simulink model "Parhuzamos_kapcsolas_szemleltetes"  (Simulink 7.6)
settings: Solver=ode45  StartTime=0.0  StopTime=10.0  RelTol=1e-3
libraries: fl_lib x17
settings Model: Creator=Fodi  LastModifiedBy=Fodi

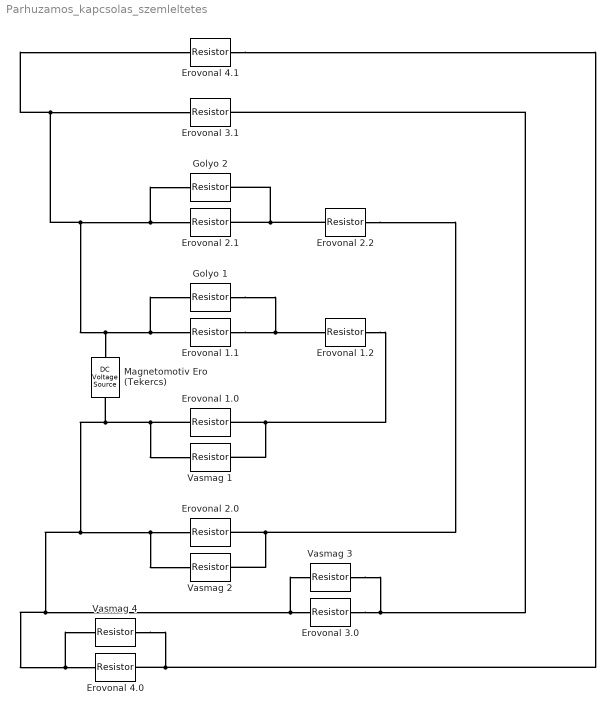
== system Parhuzamos_kapcsolas_szemleltetes ==
  Erovonal 1.0 : fl_lib/Electrical/Electrical Elements/Resistor  DialogController=NetworkEngine.DynNeDlgSource  SystemSampleTime=-1  R=1 Ohm  i_Log=off  v_Log=off  LocalVarNames=|i|v  LocalVarDescs=|i|v  LocalVarLogging=[0 0]
  Erovonal 1.1 : fl_lib/Electrical/Electrical Elements/Resistor  DialogController=NetworkEngine.DynNeDlgSource  SystemSampleTime=-1  R=1 Ohm  i_Log=off  v_Log=off  LocalVarNames=|i|v  LocalVarDescs=|i|v  LocalVarLogging=[0 0]
  Erovonal 1.2 : fl_lib/Electrical/Electrical Elements/Resistor  DialogController=NetworkEngine.DynNeDlgSource  SystemSampleTime=-1  R=1 Ohm  i_Log=off  v_Log=off  LocalVarNames=|i|v  LocalVarDescs=|i|v  LocalVarLogging=[0 0]
  Erovonal 2.0 : fl_lib/Electrical/Electrical Elements/Resistor  DialogController=NetworkEngine.DynNeDlgSource  SystemSampleTime=-1  R=1 Ohm  i_Log=off  v_Log=off  LocalVarNames=|i|v  LocalVarDescs=|i|v  LocalVarLogging=[0 0]
  Erovonal 2.1 : fl_lib/Electrical/Electrical Elements/Resistor  DialogController=NetworkEngine.DynNeDlgSource  SystemSampleTime=-1  R=1 Ohm  i_Log=off  v_Log=off  LocalVarNames=|i|v  LocalVarDescs=|i|v  LocalVarLogging=[0 0]
  Erovonal 2.2 : fl_lib/Electrical/Electrical Elements/Resistor  DialogController=NetworkEngine.DynNeDlgSource  SystemSampleTime=-1  R=1 Ohm  i_Log=off  v_Log=off  LocalVarNames=|i|v  LocalVarDescs=|i|v  LocalVarLogging=[0 0]
  Erovonal 3.0 : fl_lib/Electrical/Electrical Elements/Resistor  DialogController=NetworkEngine.DynNeDlgSource  SystemSampleTime=-1  R=1 Ohm  i_Log=off  v_Log=off  LocalVarNames=|i|v  LocalVarDescs=|i|v  LocalVarLogging=[0 0]
  Erovonal 3.1 : fl_lib/Electrical/Electrical Elements/Resistor  DialogController=NetworkEngine.DynNeDlgSource  SystemSampleTime=-1  R=1 Ohm  i_Log=off  v_Log=off  LocalVarNames=|i|v  LocalVarDescs=|i|v  LocalVarLogging=[0 0]
  Erovonal 4.0 : fl_lib/Electrical/Electrical Elements/Resistor  DialogController=NetworkEngine.DynNeDlgSource  SystemSampleTime=-1  R=1 Ohm  i_Log=off  v_Log=off  LocalVarNames=|i|v  LocalVarDescs=|i|v  LocalVarLogging=[0 0]
  Erovonal 4.1 : fl_lib/Electrical/Electrical Elements/Resistor  DialogController=NetworkEngine.DynNeDlgSource  SystemSampleTime=-1  R=1 Ohm  i_Log=off  v_Log=off  LocalVarNames=|i|v  LocalVarDescs=|i|v  LocalVarLogging=[0 0]
  Golyo 1 : fl_lib/Electrical/Electrical Elements/Resistor  DialogController=NetworkEngine.DynNeDlgSource  SystemSampleTime=-1  R=1 Ohm  i_Log=off  v_Log=off  LocalVarNames=|i|v  LocalVarDescs=|i|v  LocalVarLogging=[0 0]
  Golyo 2 : fl_lib/Electrical/Electrical Elements/Resistor  DialogController=NetworkEngine.DynNeDlgSource  SystemSampleTime=-1  R=1 Ohm  i_Log=off  v_Log=off  LocalVarNames=|i|v  LocalVarDescs=|i|v  LocalVarLogging=[0 0]
  Magnetomotiv Ero (Tekercs) : fl_lib/Electrical/Electrical Sources/DC Voltage Source  DialogController=NetworkEngine.DynNeDlgSource  SystemSampleTime=-1  v0=1 V  i_Log=off  v_Log=off  LocalVarNames=|i|v  LocalVarDescs=|i|v  LocalVarLogging=[0 0]
  Vasmag {1..4} (4 alike) : fl_lib/Electrical/Electrical Elements/Resistor  DialogController=NetworkEngine.DynNeDlgSource  SystemSampleTime=-1  R=1 Ohm  i_Log=off  v_Log=off  LocalVarNames=|i|v  LocalVarDescs=|i|v  LocalVarLogging=[0 0]
  connections:
  Golyo 1/RConn1 -- Erovonal 1.2/LConn1 -- Erovonal 1.1/RConn1
  Erovonal 2.2/LConn1 -- Erovonal 2.1/RConn1 -- Golyo 2/RConn1
  Magnetomotiv Ero (Tekercs)/LConn1 -- Erovonal 1.1/LConn1 -- Golyo 1/LConn1 -- Erovonal 3.1/LConn1 -- Erovonal 4.1/LConn1 -- Erovonal 2.1/LConn1 -- Golyo 2/LConn1
  Erovonal 1.2/RConn1 -- Erovonal 1.0/RConn1 -- Vasmag 1/RConn1
  Erovonal 2.2/RConn1 -- Erovonal 2.0/RConn1 -- Vasmag 2/RConn1
  Erovonal 1.0/LConn1 -- Vasmag 1/LConn1 -- Magnetomotiv Ero (Tekercs)/RConn1 -- Erovonal 2.0/LConn1 -- Vasmag 2/LConn1 -- Erovonal 3.0/LConn1 -- Vasmag 3/LConn1 -- Erovonal 4.0/LConn1 -- Vasmag 4/LConn1
  Erovonal 3.0/RConn1 -- Erovonal 3.1/RConn1 -- Vasmag 3/RConn1
  Erovonal 4.1/RConn1 -- Erovonal 4.0/RConn1 -- Vasmag 4/RConn1
